simulink model "cov_control_no_pinning"  (R2024a)
settings: Solver=FixedStepAuto  StartTime=0.0  StopTime=Tf  FixedStep=1  RelTol=1e-3
values from neighbouring files (symbols this model uses):
  delta = deg2rad(rand(1,n)*360/10)    [coverage1D_parameters.m]    (also in coverage_parameters.m)
  delta_bar = zeros(n,n)    [coverage1D_parameters.m]    (also in coverage_parameters.m)
  eta = 0.005.*ones(1,n)    [coverage1D_parameters.m]    (also in coverage_parameters.m)
  lambda = rand(1,n)*4.5 + ones(1,n)*0.5    [coverage1D_parameters.m]    (also in coverage_parameters.m)
  n = 5    [coverage1D_parameters.m]    (also in coverage_parameters.m)
  omega = rand(1,n)*2    [coverage1D_parameters.m]    (also in coverage_parameters.m)
  order_preservation = false    [coverage1D_parameters.m]    (also in coverage_parameters.m)
  phi = rand(1,n)*pi    [coverage1D_parameters.m]    (also in coverage_parameters.m)
  q0 = sort(rand(1, n) * 2 * pi)'    [coverage1D_parameters.m]    (also in coverage_parameters.m)
  T_star = pi/sum(lambda(1:n))    [coverage1D_parameters.m]    (also in coverage_parameters.m)
  update_step = 1    [coverage1D_parameters.m]    (also in coverage_parameters.m)
settings Model: SimulationMode=accelerator  PacingRate=10  Creator=valen  LastModifiedBy=valen

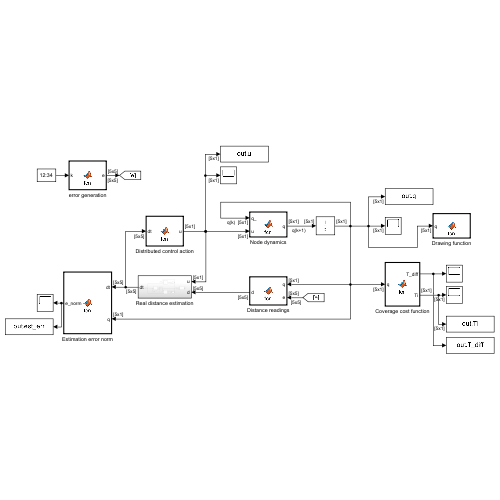
[thumbnail: Simulink's stored preview of the top-level diagram]
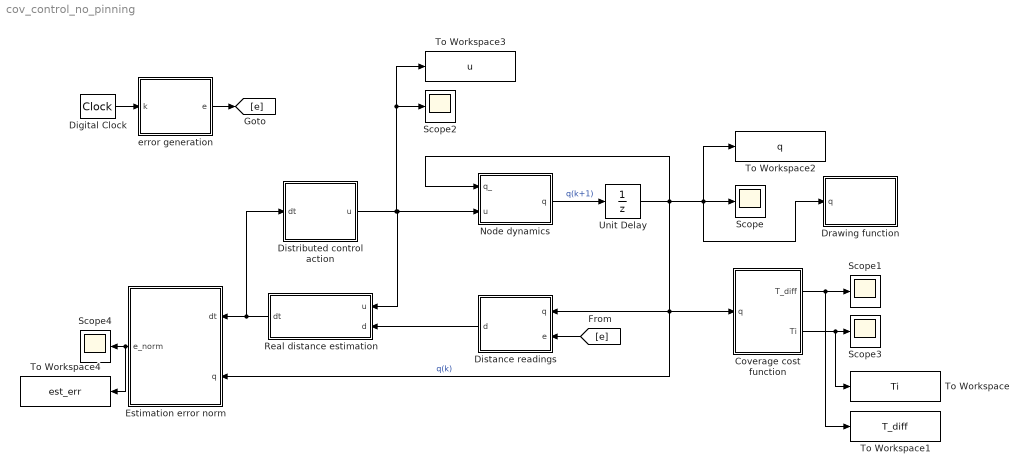
== system cov_control_no_pinning ==
  Coverage cost function : MATLAB Function  TreatAsAtomicUnit=on
  Digital Clock : DigitalClock
  Distance readings : MATLAB Function  TreatAsAtomicUnit=on
  Distributed control action : MATLAB Function  TreatAsAtomicUnit=on
  Drawing function : MATLAB Function  TreatAsAtomicUnit=on
  Estimation error norm : MATLAB Function  TreatAsAtomicUnit=on
  Node dynamics : MATLAB Function  TreatAsAtomicUnit=on
  Real distance estimation : Subsystem
  Scope{,1..4} (5 alike) : Scope
  To Workspace : ToWorkspace  VariableName=Ti  SaveFormat=Timeseries  SampleTime=-1
  To Workspace1 : ToWorkspace  VariableName=T_diff  SaveFormat=Timeseries  SampleTime=-1
  To Workspace2 : ToWorkspace  VariableName=q  SaveFormat=Timeseries  SampleTime=-1
  To Workspace3 : ToWorkspace  VariableName=u  SaveFormat=Timeseries  SampleTime=-1
  To Workspace4 : ToWorkspace  VariableName=est_err  SaveFormat=Timeseries  SampleTime=-1
  Unit Delay : UnitDelay  InitialCondition=q0  SampleTime=-1  HasFrameUpgradeWarning=on
  error generation : MATLAB Function  TreatAsAtomicUnit=on
  wires:
  Node dynamics/1(q) -> Unit Delay/1  "q(k+1)"
  Unit Delay/1 -> Node dynamics/1(q_), To Workspace2/1, Scope/1, Drawing function/1(q), Estimation error norm/2(q), Distance readings/1(q), Coverage cost function/1(q)  "q(k)"
  Digital Clock/1 -> error generation/1(k)
  [e] -> Distance readings/2(e)
  error generation/1(e) -> [e]
  Coverage cost function/1(T_diff) -> To Workspace1/1, Scope1/1
  Coverage cost function/2(Ti) -> To Workspace/1, Scope3/1
  Distributed control action/1(u) -> To Workspace3/1, Scope2/1, Node dynamics/2(u), Real distance estimation/1(u)
  Real distance estimation/1(dt) -> Distributed control action/1(dt), Estimation error norm/1(dt)
  Estimation error norm/1(e_norm) -> To Workspace4/1, Scope4/1
  Distance readings/1(d) -> Real distance estimation/2(d)

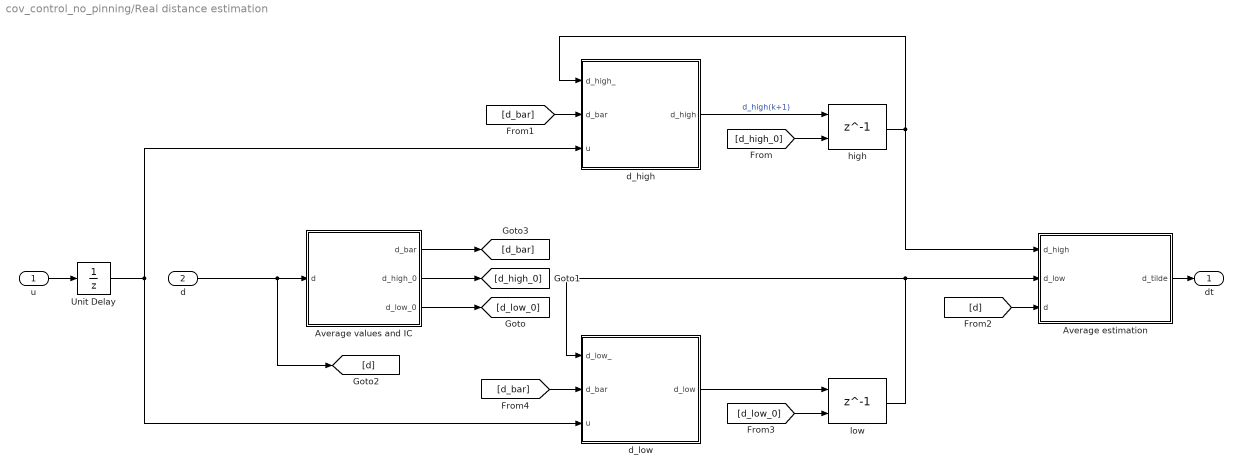
== system cov_control_no_pinning/Real distance estimation ==
  u : Inport
  d : Inport  Port=2
  Average estimation : MATLAB Function  TreatAsAtomicUnit=on
  Average values and IC : MATLAB Function  TreatAsAtomicUnit=on
  Unit Delay : UnitDelay  SampleTime=-1  HasFrameUpgradeWarning=on
  d_high : MATLAB Function  TreatAsAtomicUnit=on
  d_low : MATLAB Function  TreatAsAtomicUnit=on
  high : Delay  DelayLength=1  InitialConditionSource=Input port
      settings: InputPortMap=u0,p4
  low : Delay  DelayLength=1  InitialConditionSource=Input port
      settings: InputPortMap=u0,p4
  dt : Outport
  wires:
  d_high/1(d_high) -> high/1  "d_high(k+1)"
  d/1 -> Average values and IC/1(d), [d]
  high/1 -> d_high/1(d_high_), Average estimation/1(d_high)
  Average values and IC/3(d_low_0) -> [d_low_0]
  Average values and IC/2(d_high_0) -> [d_high_0]
  [d_high_0] -> high/2
  Average values and IC/1(d_bar) -> [d_bar]
  [d_bar] -> d_high/2(d_bar)
  [d_low_0] -> low/2
  low/1 -> Average estimation/2(d_low), d_low/1(d_low_)
  d_low/1(d_low) -> low/1
  [d_bar] -> d_low/2(d_bar)
  Average estimation/1(d_tilde) -> dt/1
  [d] -> Average estimation/3(d)
  u/1 -> Unit Delay/1
  Unit Delay/1 -> d_high/3(u), d_low/3(u)

== matlab function cov_control_no_pinning/Real distance estimation/d_high ==
  data: d_high_ input; d_bar input; u input; d_high output; delta_bar parameter; n parameter
function d_high = fcn(d_high_, d_bar, u, delta_bar,n)

    d_high = zeros(n,n);

    for i=1:n
        j = previous_i(i,n);
        d_high(i,j) = min([d_bar(i,j) + delta_bar(i,j); d_high_(i,j) + u(j) - u(i)]);

        j = next_i(i,n);
        d_high(i,j) = min([d_bar(i,j) + delta_bar(i,j); d_high_(i,j) + u(j) - u(i)]);
    end

== matlab function cov_control_no_pinning/Real distance estimation/d_low ==
  data: d_low_ input; d_bar input; u input; d_low output; delta_bar parameter; n parameter
function d_low = fcn(d_low_, d_bar, u, delta_bar,n)

    d_low = zeros(n,n);

    for i=1:n
        j = previous_i(i,n);
        d_low(i,j) = max([d_bar(i,j) - delta_bar(i,j); d_low_(i,j) + u(j) - u(i)]);

        j = next_i(i,n);
        d_low(i,j) = max([d_bar(i,j) - delta_bar(i,j); d_low_(i,j) + u(j) - u(i)]);
    end

== matlab function cov_control_no_pinning/Distributed control action ==
  data: dt input; u output size=[n,1]; eta parameter; lambda parameter; n parameter; order_preservation parameter
function u = fcn(dt, eta, lambda,n,order_preservation)
    ut = zeros(n,1);
    for i=1:n

        ut(i) = eta(i)*( ...
                (lambda(previous_i(i,n)) + lambda(i))*dt(i, next_i(i,n)) + ...
                (lambda(i) + lambda(next_i(i,n)))*dt(i,previous_i(i,n))...
                );
    end

    % saturation of u_tilde
    if order_preservation
        u = lambda'.*max(min(ut, 1), 0);
    else
        u = lambda'.*max(min(ut, 1), -1);
    end

== matlab function cov_control_no_pinning/Node dynamics ==
  data: q_ input; u input; q output
function q = fcn(q_, u)

    q = (q_ + u);

== matlab function cov_control_no_pinning/error generation ==
  data: k input; e output size=[n,n]; omega parameter; phi parameter; delta parameter; n parameter
function e = fcn(k,omega, phi, delta,n)
    e = zeros(n,n);

    for i=1:n
        j = previous_i(i,n);
        e(i,j) = (1+3*sin(omega(i)*k + 10*(j-i)*phi(i)))*delta(i)/4;

        j = next_i(i,n);
        e(i,j) = (1+3*sin(omega(i)*k + 10*(j-i)*phi(i)))*delta(i)/4;    
    end

== matlab function cov_control_no_pinning/Distance readings ==
  data: q input; d output; e input; n parameter; update_step parameter
function d = fcn(q,e,n,update_step)
        
        persistent counter;
        persistent last_d;
        
        if isempty(counter)
            counter = 1;
        end
        if isempty(last_d)
            last_d = zeros(n,n);
        end

        counter = counter + 1;

        if mod(counter,update_step) == 0
       
            for i=1:n
            
                j = previous_i(i,n);
                last_d(i, j) = compute_distance(q(i),q(j), "previous") + e(i,j);
        
                j = next_i(i,n);
                last_d(i, j) = compute_distance(q(i),q(j), "next") + e(i,j);
            end
        end

        d = last_d;


end

== matlab function cov_control_no_pinning/Estimation error norm ==
  data: dt input; e_norm output; q input; n parameter
function e_norm = fcn(dt, q, n)

    real_distance = zeros(n,n);

    for i=1:n
        
        j = previous_i(i,n);
        real_distance(i, j) = -circular_distance(q(i), q(j));

        j = next_i(i,n);
        real_distance(i, j) = circular_distance(q(i), q(j));
    end

    e_norm=norm(real_distance-dt);

== matlab function cov_control_no_pinning/Coverage cost function ==
  data: q input; T_diff output; lambda parameter; T_star parameter; Ti output; n parameter
function [T_diff, Ti] = fcn(q, lambda, T_star, n)


    max_min_time = -Inf;

    for s = linspace(0,2*pi,1000)
        min_time = Inf;

        for i=1:n

            arrival_time = (circular_distance(q(i),s))/lambda(i);
            if(arrival_time < min_time)
                min_time = arrival_time;
            end

        end

        if(min_time > max_min_time)
            max_min_time = min_time;
        end

    end

    T = max_min_time;
    T_diff = T - T_star;

    Ti = zeros(n,1);
    for i=1:n
       Ti(i) = compute_distance(q(i), q(next_i(i,n)), "next")/(lambda(i) + lambda(next_i(i,n))); 
    end

== matlab function cov_control_no_pinning/Drawing function ==
  data: q input
function fcn(q)

    x = cos(q);
    y = sin(q);

    persistent h;
    if isempty(h)
        figure;
        h = plot(x, y, 'ro');
        axis equal;
        axis([-1.5 1.5 -1.5 1.5]);
        grid on;
    else
        set(h, 'XData', x, 'YData', y);
        drawnow;
    end

== matlab function cov_control_no_pinning/Real distance estimation/Average estimation ==
  data: d_high input; d_tilde output; d_low input; d input; n parameter
function d_tilde = fcn(d_high, d_low, d, n)

    d_tilde = (d_high + d_low)/2;
    
    for i=1:n
    
        j = next_i(i,n);
        if d_high(i,j)<d_low(i,j)
            d_tilde(i,j) = d(i,j);
        end
    
        j = previous_i(i,n);
        if d_high(i,j)<d_low(i,j)
            d_tilde(i,j) = d(i,j);
        end
    
        
    end

== matlab function cov_control_no_pinning/Real distance estimation/Average values and IC ==
  data: d input; d_bar output; delta_bar parameter; d_high_0 output; d_low_0 output
function [d_bar, d_high_0, d_low_0] = fcn(d,delta_bar)

    
    d_bar = (d - d')/2; 

    persistent flag;
    persistent dh0;
    persistent dl0;
    
    if isempty(flag)
        
        d_high_0 = d_bar + delta_bar;
        d_low_0 = d_bar - delta_bar;
        
        dh0 = d_high_0;
        dl0 = d_low_0;
        
        flag=1;
    else
        d_high_0 = dh0;
        d_low_0 = dl0;
    end
